simulink library "tp81559a4b_14bf_4325_96d3_99db43361ac9"  (Simulink 7.0)
settings Model: Creator=fo1521  LastModifiedBy=fo1521

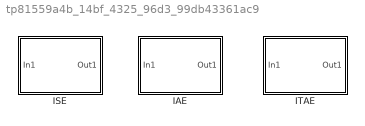
== system tp81559a4b_14bf_4325_96d3_99db43361ac9 ==
  IAE : Subsystem
      mask Description:
      | IAE performacne index
      | 
      | output = int |input| dt
      mask Display:
      | disp('IAE')
      | port_label('input',1,'e')
      | port_label('output',1,'iae')
  ISE : Subsystem
      mask Description:
      | ISE performance index
      | 
      | output = int (input)^2 dt
      mask Display:
      | disp('ISE')
      | port_label('input',1,'e')
      | port_label('output',1,'ise')
  ITAE : Subsystem
      mask Description:
      | ITAE performance index
      | 
      | output = int t|input| dt
      mask Display:
      | disp('ITAE')
      | port_label('input',1,'e')
      | port_label('output',1,'itae')

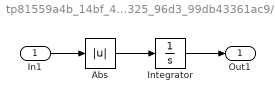
== system tp81559a4b_14bf_4325_96d3_99db43361ac9/IAE ==
  In1 : Inport
  Abs : Abs
  Integrator : Integrator
  Out1 : Outport
  wires:
  Abs/1 -> Integrator/1
  Integrator/1 -> Out1/1
  In1/1 -> Abs/1

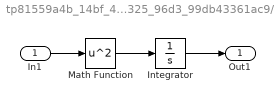
== system tp81559a4b_14bf_4325_96d3_99db43361ac9/ISE ==
  In1 : Inport
  Integrator : Integrator
  Math Function : Math  Operator=square  OutDataType=sfix(16)  OutScaling=2^0  SaturateOnIntegerOverflow=on
  Out1 : Outport
  wires:
  In1/1 -> Math Function/1
  Integrator/1 -> Out1/1
  Math Function/1 -> Integrator/1

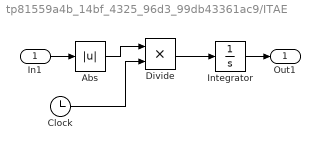
== system tp81559a4b_14bf_4325_96d3_99db43361ac9/ITAE ==
  In1 : Inport
  Abs : Abs
  Clock : Clock
      settings: Decimation=10
  Divide : Product  Inputs=**  OutDataType=sfix(16)  OutScaling=2^-10
  Integrator : Integrator
  Out1 : Outport
  wires:
  Clock/1 -> Divide/2
  Abs/1 -> Divide/1
  Divide/1 -> Integrator/1
  In1/1 -> Abs/1
  Integrator/1 -> Out1/1
